simulink model "caso_scalare_con_ingresso"  (R2024b)
settings: Solver=VariableStepAuto  StartTime=0.0  StopTime=25.0  RelTol=1e-3
settings Model: Creator=david  LastModifiedBy=david

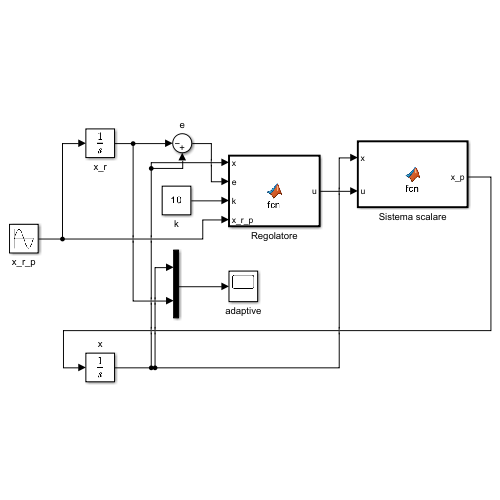
[thumbnail: Simulink's stored preview of the top-level diagram]
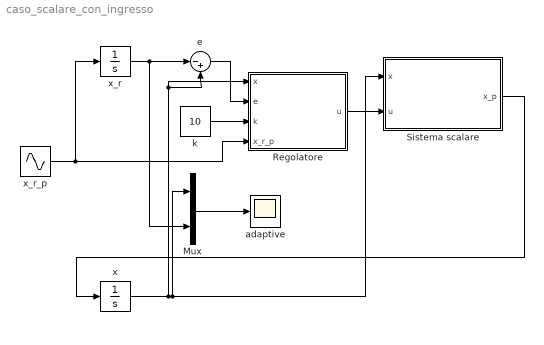
== system caso_scalare_con_ingresso ==
  Mux : Mux  Inputs=2
  Regolatore : MATLAB Function  TreatAsAtomicUnit=on
  Sistema scalare : MATLAB Function  TreatAsAtomicUnit=on
  adaptive : Scope
  e : Sum  Inputs=|-+
  k : Constant  Value=10  VectorParams1D=off
  x : Integrator  InitialCondition=1
  x_r : Integrator
  x_r_p : Sin  Phase=90  SampleTime=0
  wires:
  k/1 -> Regolatore/3(k)
  x_r_p/1 -> Regolatore/4(x_r_p), x_r/1
  e/1 -> Regolatore/2(e)
  x_r/1 -> Mux/2, e/1
  Sistema scalare/1(x_p) -> x/1
  x/1 -> Sistema scalare/1(x), Mux/1, Regolatore/1(x), e/2
  Mux/1 -> adaptive/1
  Regolatore/1(u) -> Sistema scalare/2(u)

== matlab function caso_scalare_con_ingresso/Regolatore ==
  data: x input; u output; e input; k input; x_r_p input
function u = fcn(x,e,k,x_r_p)

a = 1;
u = -a*x + x_r_p -k*e;%regolazione

== matlab function caso_scalare_con_ingresso/Sistema scalare ==
  data: x input; x_p output; u input
function x_p = fcn(x,u)

a = 1;
x_p = a*x + u;
